simulink model "AME552_HW2_P3_SimulinkModel"  (R2024b)
settings: Solver=VariableStepAuto  StartTime=0.0  StopTime=5  RelTol=1e-3
values from neighbouring files (symbols this model uses):
  de0 = de0_space(j)    [AME552_HW2_P3_Simulink.m]
  e0 = e0_space(i)    [AME552_HW2_P3_Simulink.m]
libraries: simulink x1
settings Model: Creator=lewis  LastModifiedBy=lewis

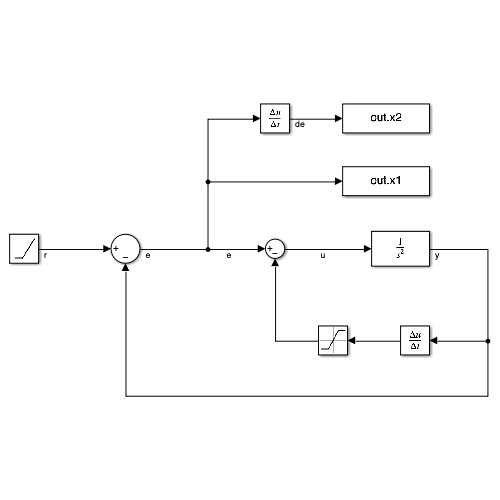
[thumbnail: Simulink's stored preview of the top-level diagram]
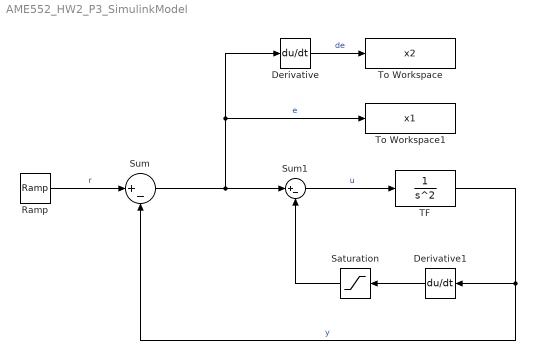
== system AME552_HW2_P3_SimulinkModel ==
  Derivative : Derivative
  Derivative1 : Derivative
  Ramp : simulink/Sources/Ramp  slope=de0  start=0  InitialOutput=e0
  Saturation : Saturate  UpperLimit=1  LowerLimit=-1
  Sum : Sum  Inputs=|+-
  Sum1 : Sum  Inputs=|+-
  TF : TransferFcn  Denominator=[1 0 0]
  To Workspace : ToWorkspace  VariableName=x2  SaveFormat=Timeseries  SampleTime=-1
  To Workspace1 : ToWorkspace  VariableName=x1  SaveFormat=Timeseries  SampleTime=-1
  wires:
  Sum/1 -> Sum1/1, To Workspace1/1, Derivative/1  "e"
  TF/1 -> Sum/2, Derivative1/1  "y"
  Derivative/1 -> To Workspace/1  "de"
  Sum1/1 -> TF/1  "u"
  Derivative1/1 -> Saturation/1
  Saturation/1 -> Sum1/2
  Ramp/1 -> Sum/1  "r"
